simulink model "blockdemo"  (Simulink 6.3)
settings: Solver=VariableStepDiscrete  StartTime=0.0  StopTime=20  FixedStep=1  RelTol=1e-3
InitFcn:
  | %% DSPBuilder Start
  | alt_dspbuilder_update_model(bdroot)
  | %% DSPBuilder End
libraries: allblocks_alteradspbuilder2 x9
settings Model: Creator=mjervis  LastModifiedBy=delphick
settings OptimizationCC: BlockReduction=off  BooleanDataType=off  InlineInvariantSignals=on
settings DebuggingCC: SolverPrmCheckMsg=none
settings HardwareCC: TargetUnknown=on

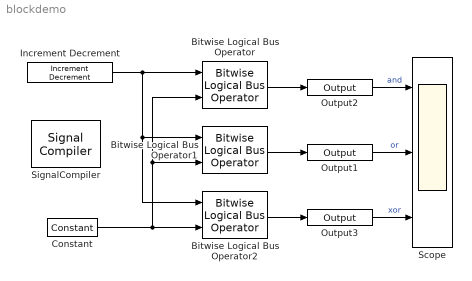
== system blockdemo ==
  Bitwise Logical Bus Operator : allblocks_alteradspbuilder2/Bitwise Logical Bus Operator  BusType=Inferred  bwl=4  bwr=0  LogicalOperator=AND
  Bitwise Logical Bus Operator1 : allblocks_alteradspbuilder2/Bitwise Logical Bus Operator  BusType=Inferred  bwl=8  bwr=0  LogicalOperator=OR
  Bitwise Logical Bus Operator2 : allblocks_alteradspbuilder2/Bitwise Logical Bus Operator  BusType=Inferred  bwl=8  bwr=0  LogicalOperator=XOR
  Constant : allblocks_alteradspbuilder2/Constant  mask_cst=3  BusType=Signed Integer  bwl=4  bwr=0  SpecifyClock=off
  Increment Decrement : allblocks_alteradspbuilder2/Increment Decrement  BusType=Unsigned Integer  bwl=4  bwr=8  SpecifyClock=off  clr_value=0  direction=Increment  phase_selection=1  use_ena=off  use_sclr=off
  Output1 : allblocks_alteradspbuilder2/Output  iofile=C:\workspace_clean\Documentation\DesignExamples\Tutorials\UnitBlocks\GateAndControl\BitwiseLogicalBusOperator\tb_blockdemo\blockdemo_Output1.capture  BusType=Unsigned Integer  bwl=4  bwr=0  PORTTYPE=Output
  Output2 : allblocks_alteradspbuilder2/Output  iofile=C:\workspace_clean\Documentation\DesignExamples\Tutorials\UnitBlocks\GateAndControl\BitwiseLogicalBusOperator\tb_blockdemo\blockdemo_Output2.capture  BusType=Unsigned Integer  bwl=4  bwr=0  PORTTYPE=Output
  Output3 : allblocks_alteradspbuilder2/Output  iofile=C:\workspace_clean\Documentation\DesignExamples\Tutorials\UnitBlocks\GateAndControl\BitwiseLogicalBusOperator\tb_blockdemo\blockdemo_Output3.capture  BusType=Unsigned Integer  bwl=4  bwr=0  PORTTYPE=Output
  Scope : Scope  NumInputPorts=3
      settings: TimeRange=20  YMin=-1~0~0  YMax=4~20~20
  SignalCompiler : allblocks_alteradspbuilder2/Signal Compiler  DeviceFamily=Stratix III  DeviceName=AUTO  EnableSignalTap=off  SignalTapDepth=128  UseBoardBlock=off  StpUseDefaultClock=on  StpClock=clock
  wires:
  Output1/1 -> Scope/2  "or"
  Output2/1 -> Scope/1  "and"
  Increment Decrement/1 -> Bitwise Logical Bus Operator/1, Bitwise Logical Bus Operator2/1, Bitwise Logical Bus Operator1/1
  Constant/1 -> Bitwise Logical Bus Operator2/2, Bitwise Logical Bus Operator1/2, Bitwise Logical Bus Operator/2
  Bitwise Logical Bus Operator/1 -> Output2/1
  Bitwise Logical Bus Operator1/1 -> Output1/1
  Bitwise Logical Bus Operator2/1 -> Output3/1
  Output3/1 -> Scope/3  "xor"
